simulink model "levitron_xpc"  (Simulink 7.1)
settings: Solver=ode4  StartTime=0.0  StopTime=inf  FixedStep=0.01  RelTol=1e-3
libraries: xpclib x4, xpcutilitieslib x2, levitron_lib x1
settings Model: Creator=volgy  LastModifiedBy=volgy  BufferReuse=off
settings OptimizationCC: BlockReduction=off  OptimizeBlockIOStorage=off  BufferReuse=off  ExpressionFolding=off  LocalBlockOutputs=off
settings HardwareCC: ProdIntDivRoundTo=Zero  ProdEndianess=LittleEndian  ProdHWDeviceType=Generic->32-bit x86 compatible
settings RTWCC: SystemTargetFile=xpctarget.tlc  TemplateMakefile=xpc_default_tmf  Description=xPC Target  ProcessScript=xpctarget_make_rtw_hook
settings xpcTargetCC: TargetFcnLib=ansi_tfl_table_tmw.mat  TargetFunctionLibrary=ANSI_C  CompOptLevelCompliant=off  PortableWordSizes=off  xPCisDownloadable=off

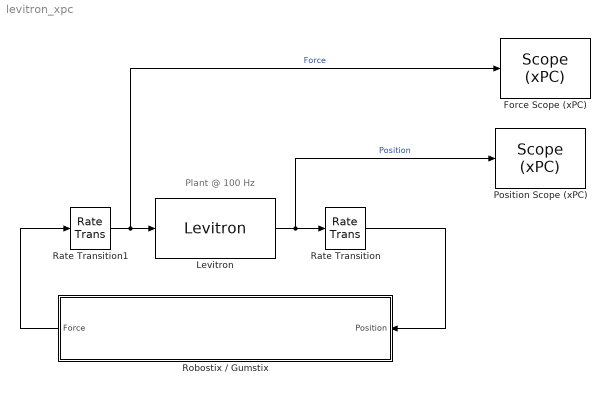
== system levitron_xpc ==
  note: Plant @ 100 Hz
  Force Scope (xPC) : xpclib/Misc./Scope (xPC)   SystemSampleTime=-1  scopeno=2  scopetype=Target  autostart=on  viewmode=Graphical sliding  formatstr='%15.6f'  grid=on  ylimits=[0,0]  nosamples=10000  noprepostsamples=0  interleave=1  triggermode=FreeRun  triggersignal=1  triggerlevel=0.0  triggerslope=Either  triggerscope=1  triggersample=0  filename=data.dat  mode=Lazy  writesize=512  autorestart=off
  Levitron : levitron_lib/Levitron  SystemSampleTime=-1  mass=1  gravity=-9.81  v0=15  z0=10
  "Position Scope (xPC) " : xpclib/Misc./Scope (xPC)   SystemSampleTime=-1  scopeno=1  scopetype=Target  autostart=on  viewmode=Graphical sliding  formatstr='%15.6f'  grid=on  ylimits=[0,0]  nosamples=10000  noprepostsamples=0  interleave=1  triggermode=FreeRun  triggersignal=1  triggerlevel=0.0  triggerslope=Either  triggerscope=1  triggersample=0  filename=data.dat  mode=Lazy  writesize=512  autorestart=off
  Rate Transition : RateTransition  OutPortSampleTime=0.02
  Rate Transition1 : RateTransition  OutPortSampleTime=0.01
  Robostix / Gumstix : Subsystem  Orientation=left
  wires:
  Rate Transition1/1 -> Levitron/1, Force Scope (xPC)/1  "Force"
  Levitron/1 -> Rate Transition/1, "Position Scope (xPC) "/1  "Position"
  Rate Transition/1 -> Robostix / Gumstix/1(Position)
  Robostix / Gumstix/1(Force) -> Rate Transition1/1

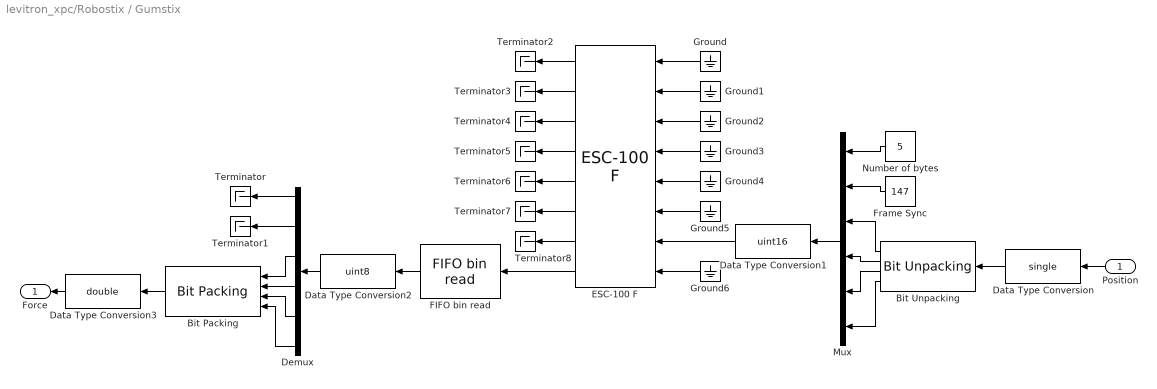
== system levitron_xpc/Robostix / Gumstix ==
  Position : Inport  Orientation=left
  "Bit Packing " : xpcutilitieslib/Bit Packing   Orientation=left  MaskBitPatterns={[0:7], [8:15], [16:23], [24:31]}  MaskPackDataType=single  MaskPackDataSize=[1]
  "Bit Unpacking " : xpcutilitieslib/Bit Unpacking   Orientation=left  SignExtend=off  MaskBitPatterns={[0:7], [8:15], [16:23], [24:31]}  MaskPackDataType=single  MaskPackDataSize=[1]  MaskUnpackDataTypes={'uint8', 'uint8', 'uint8', 'uint8'}  MaskUnpackDataSizes={[1], [1], [1], [1]}
  Data Type Conversion : DataTypeConversion  Orientation=left  OutDataTypeMode=single  OutDataType=sfix(16)  OutScaling=2^0  OutDataTypeStr=single
  Data Type Conversion1 : DataTypeConversion  Orientation=left  OutDataTypeMode=uint16  OutDataType=sfix(16)  OutScaling=2^0  OutDataTypeStr=uint16  ConvertRealWorld=Stored Integer (SI)
  Data Type Conversion2 : DataTypeConversion  Orientation=left  OutDataTypeMode=uint8  OutDataType=sfix(16)  OutScaling=2^0  OutDataTypeStr=uint8
  Data Type Conversion3 : DataTypeConversion  Orientation=left  OutDataTypeMode=double  OutDataType=sfix(16)  OutScaling=2^0  OutDataTypeStr=double
  Demux : Demux  Orientation=left  Outputs=6
  ESC-100 F : xpclib/RS232/Quatech/ESC-100/ESC-100 F  Orientation=left  SystemSampleTime=-1  group=Basic Setup  port=1  irqnum=10  slot=-1  baud1=57600  parity1=None  ndata1=8  nstop1=1  fifomode1=64 deep  rlevel1=half full  automode1=off  xmtfifosize1=1024  xmtdatatype1=count+16 bit uint  rcvfifosize1=1024  baud2=57600  parity2=None  ndata2=8  nstop2=1  fifomode2=64 deep  rlevel2=half full  automode2=off  xmtfifosize2=1024  xmtdatatype2=count+16 bit uint  rcvfifosize2=1024  baud3=57600  parity3=None  ndata3=8  nstop3=1  fifomode3=64 deep  rlevel3=half full  automode3=off  xmtfifosize3=1024  xmtdatatype3=count+16 bit uint  rcvfifosize3=1024  buad4=57600  parity4=None  ndata4=8  nstop4=1  fifomode4=64 deep  rlevel4=half full  automode4=off  xmtfifosize4=1024  xmtdatatype4=count+16 bit uint  rcvfifosize4=1024  baud5=57600  parity5=None  ndata5=8  nstop5=1  fifomode5=64 deep  rlevel5=half full  automode5=off  xmtfifosize5=1024  xmtdatatype5=count+16 bit uint  rcvfifosize5=1024  baud6=57600  parity6=None  ndata6=8  nstop6=1  fifomode6=64 deep  rlevel6=half full  automode6=off  xmtfifosize6=1024  xmtdatatype6=count+16 bit uint  rcvfifosize6=1024  baud7=57600  parity7=None  ndata7=8  nstop7=1  fifomode7=64 deep  rlevel7=half full  automode7=off  xmtfifosize7=1024  xmtdatatype7=count+16 bit uint  rcvfifosize7=1024  baud8=57600  parity8=None  ndata8=8  nstop8=1  fifomode8=64 deep  rlevel8=half full  automode8=off  xmtfifosize8=1024  xmtdatatype8=count+16 bit uint  rcvfifosize8=1024
  FIFO bin read : xpclib/RS232/FIFO bin read   Orientation=left  header={char([147])}  lengths=[5]  hold=Zero output if no new data  enable=off  maxsize=5  outputtype=count+16 bit uint  sampletime=-1
  Frame Sync : Constant  Orientation=left  Value=147  OutDataTypeMode=uint8  OutDataType=sfix(16)  OutScaling=2^0  OutDataTypeStr=uint8
  Ground{,1..6} (7 alike) : Ground  Orientation=left
  Mux : Mux  Orientation=left  Inputs=6
  Number of bytes : Constant  Orientation=left  Value=5  OutDataTypeMode=uint8  OutDataType=sfix(16)  OutScaling=2^0  OutDataTypeStr=uint8
  Terminator{,1..8} (9 alike) : Terminator
  Force : Outport  Orientation=left
  wires:
  Data Type Conversion/1 -> "Bit Unpacking "/1
  "Bit Unpacking "/4 -> Mux/6
  "Bit Unpacking "/3 -> Mux/5
  "Bit Unpacking "/2 -> Mux/4
  "Bit Unpacking "/1 -> Mux/3
  Frame Sync/1 -> Mux/2
  Number of bytes/1 -> Mux/1
  Mux/1 -> Data Type Conversion1/1
  Data Type Conversion1/1 -> ESC-100 F/7
  FIFO bin read/1 -> Data Type Conversion2/1
  Demux/1 -> Terminator/1
  Demux/2 -> Terminator1/1
  Demux/3 -> "Bit Packing "/1
  Demux/4 -> "Bit Packing "/2
  Demux/5 -> "Bit Packing "/3
  Demux/6 -> "Bit Packing "/4
  "Bit Packing "/1 -> Data Type Conversion3/1
  ESC-100 F/1 -> Terminator2/1
  ESC-100 F/2 -> Terminator3/1
  ESC-100 F/3 -> Terminator4/1
  ESC-100 F/4 -> Terminator5/1
  ESC-100 F/5 -> Terminator6/1
  ESC-100 F/6 -> Terminator7/1
  ESC-100 F/7 -> Terminator8/1
  Ground/1 -> ESC-100 F/1
  Ground1/1 -> ESC-100 F/2
  Ground2/1 -> ESC-100 F/3
  Ground3/1 -> ESC-100 F/4
  Ground4/1 -> ESC-100 F/5
  Ground5/1 -> ESC-100 F/6
  Ground6/1 -> ESC-100 F/8
  ESC-100 F/8 -> FIFO bin read/1
  Position/1 -> Data Type Conversion/1
  Data Type Conversion3/1 -> Force/1
  Data Type Conversion2/1 -> Demux/1
